simulink model "Winda_2015b"  (R2015b)
settings: Solver=FixedStepDiscrete  StartTime=0.0  StopTime=100  FixedStep=0.05  MaxStep=0.1  MinStep=0.01  RelTol=1e-3
undefined symbols (not defined in the file): sigbuilder_block
libraries: simulink x12
settings Model: Creator=dmar  LastModifiedBy=lab
settings DataIOCC: SaveFormat=Array  SignalLoggingSaveFormat=ModelDataLogs
settings OptimizationCC: ExpressionDepthLimit=2147483647
settings DebuggingCC: UnderspecifiedInitializationDetection=Classic  MergeDetectMultiDrivingBlocksExec=none  SolverPrmCheckMsg=warning  ParameterPrecisionLossMsg=none  FcnCallInpInsideContextMsg=UseLocalSettings  StateNameClashWarn=warning
settings HardwareCC: ProdBitPerPointer=32  ProdLargestAtomicFloat=None  ProdIntDivRoundTo=Undefined  ProdEndianess=Unspecified  ProdWordSize=32  ProdHWDeviceType=32-bit Generic
settings SFSimCC: SimParseCustomCode=off
settings GRTTargetCC: GeneratePreprocessorConditionals=Disable all  CombineOutputUpdateFcns=off  GRTInterface=on
settings ConfigComp: CovModelRefEnable=Off

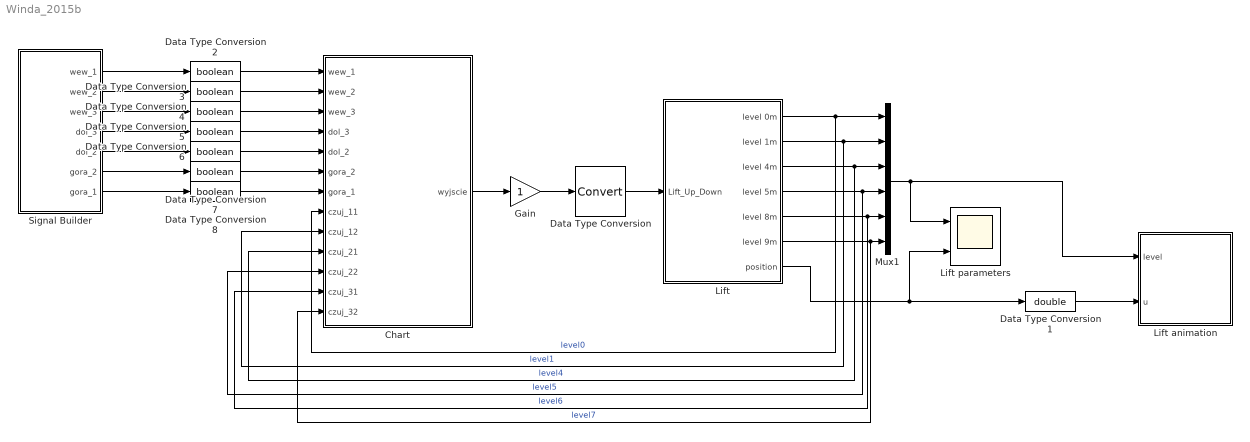
== system Winda_2015b ==
  Chart : Stateflow chart  TreatAsAtomicUnit=on
  Data Type Conversion : DataTypeConversion
  Data Type Conversion1 : DataTypeConversion  OutDataTypeStr=double
  Data Type Conversion{2..8} (7 alike) : DataTypeConversion  OutDataTypeStr=boolean
  Gain : Gain
  Lift : Subsystem
  Lift animation : MATLAB Function  TreatAsAtomicUnit=on  SystemSampleTime=0.05
  Lift parameters : Scope  NumInputPorts=2
  Mux1 : Mux  Inputs=6
  Signal Builder : Subsystem  Tag=STV Subsys  LoadFcn=sigbuilder_block('load',[81 111.75 550.5 630.75 ]);  StartFcn=sigbuilder_block('start');  StopFcn=sigbuilder_block('stop');  ClipboardFcn=sigbuilder_block('clipboard');  mask(Sigbuilder block){}
      mask help: Simulink:masks:SigbuilderBlock_MD
      mask init:
      | if ~strcmp(get_param(bdroot(gcbh),'SimulationStatus'),'stopped') tuvar = sigbuilder_block('maskInit'); end
      settings: CopyFcn=sigbuilder_block('copy');  DeleteFcn=sigbuilder_block('delete');  ModelCloseFcn=sigbuilder_block('modelClose');  PreSaveFcn=sigbuilder_block('preSave');  PauseFcn=sigbuilder_block('pause');  ContinueFcn=sigbuilder_block('continue');  NameChangeFcn=sigbuilder_block('namechange');  OpenFcn=sigbuilder_block('open',[81 111.75 550.5 630.75 ]);  CloseFcn=sigbuilder_block('close');
      mask Display: plot(0, 0, 100, 100,[2, 2, 32, 32, 2], [68, 8, 8, 68, 68],[32, 2], [38, 38], [32, 19, 2],[53, 60, 44], [32, 17, 17, 2],[16, 16, 31, 31]);txt = getActiveGroup(gcbh);text(2, 100, txt,'verticalAlignment', 'top');
  wires:
  Lift/7(position) -> Lift parameters/2, Data Type Conversion1/1
  Gain/1 -> Data Type Conversion/1
  Mux1/1 -> Lift parameters/1, Lift animation/1(level)
  Lift/1(level 0m) -> Chart/8(czuj_11), Mux1/1  "level0"
  Lift/2(level 1m) -> Chart/9(czuj_12), Mux1/2  "level1"
  Lift/3(level 4m) -> Chart/10(czuj_21), Mux1/3  "level4"
  Lift/4(level 5m) -> Chart/11(czuj_22), Mux1/4  "level5"
  Lift/5(level 8m) -> Mux1/5, Chart/12(czuj_31)  "level6"
  Lift/6(level 9m) -> Mux1/6, Chart/13(czuj_32)  "level7"
  Data Type Conversion/1 -> Lift/1(Lift_Up_Down)
  Data Type Conversion1/1 -> Lift animation/2(u)
  Chart/1(wyjscie) -> Gain/1
  Signal Builder/2(wew_2) -> Data Type Conversion3/1
  Signal Builder/3(wew_3) -> Data Type Conversion4/1
  Signal Builder/4(dol_3) -> Data Type Conversion5/1
  Signal Builder/5(dol_2) -> Data Type Conversion6/1
  Signal Builder/6(gora_2) -> Data Type Conversion7/1
  Signal Builder/7(gora_1) -> Data Type Conversion8/1
  Signal Builder/1(wew_1) -> Data Type Conversion2/1
  Data Type Conversion2/1 -> Chart/1(wew_1)
  Data Type Conversion3/1 -> Chart/2(wew_2)
  Data Type Conversion4/1 -> Chart/3(wew_3)
  Data Type Conversion5/1 -> Chart/4(dol_3)
  Data Type Conversion6/1 -> Chart/5(dol_2)
  Data Type Conversion7/1 -> Chart/6(gora_2)
  Data Type Conversion8/1 -> Chart/7(gora_1)

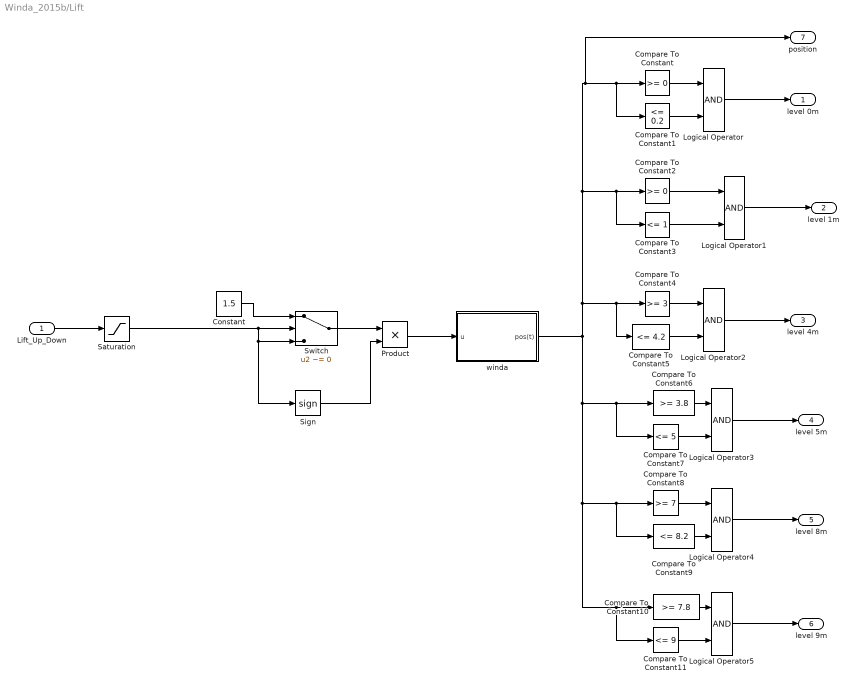
== system Winda_2015b/Lift ==
  Lift_Up_Down : Inport
  Compare To Constant : simulink/Logic and Bit Operations/Compare To Constant  relop=>=  const=0  OutDataTypeStr=boolean
  Compare To Constant1 : simulink/Logic and Bit Operations/Compare To Constant  relop=<=  const=0.2  OutDataTypeStr=boolean
  Compare To Constant10 : simulink/Logic and Bit Operations/Compare To Constant  relop=>=  const=7.8  OutDataTypeStr=boolean
  Compare To Constant11 : simulink/Logic and Bit Operations/Compare To Constant  relop=<=  const=9  OutDataTypeStr=boolean
  Compare To Constant2 : simulink/Logic and Bit Operations/Compare To Constant  relop=>=  const=0  OutDataTypeStr=boolean
  Compare To Constant3 : simulink/Logic and Bit Operations/Compare To Constant  relop=<=  const=1  OutDataTypeStr=boolean
  Compare To Constant4 : simulink/Logic and Bit Operations/Compare To Constant  relop=>=  const=3  OutDataTypeStr=boolean
  Compare To Constant5 : simulink/Logic and Bit Operations/Compare To Constant  relop=<=  const=4.2  OutDataTypeStr=boolean
  Compare To Constant6 : simulink/Logic and Bit Operations/Compare To Constant  relop=>=  const=3.8  OutDataTypeStr=boolean
  Compare To Constant7 : simulink/Logic and Bit Operations/Compare To Constant  relop=<=  const=5  OutDataTypeStr=boolean
  Compare To Constant8 : simulink/Logic and Bit Operations/Compare To Constant  relop=>=  const=7  OutDataTypeStr=boolean
  Compare To Constant9 : simulink/Logic and Bit Operations/Compare To Constant  relop=<=  const=8.2  OutDataTypeStr=boolean
  Constant : Constant  Value=1.5
  Logical Operator{,1..5} (6 alike) : Logic  AllPortsSameDT=off  OutDataTypeStr=boolean
  Product : Product  OutDataTypeStr=Inherit: Inherit via back propagation  RndMeth=Zero
  Saturation : Saturate  UpperLimit=1  LowerLimit=-1
  Sign : Signum
  Switch : Switch  Criteria=u2 ~= 0  OutDataTypeStr=Inherit: Inherit via back propagation
  winda : Subsystem
  level 0m : Outport
  level 1m : Outport  Port=2
  level 4m : Outport  Port=3
  level 5m : Outport  Port=4
  level 8m : Outport  Port=5
  level 9m : Outport  Port=6
  position : Outport  Port=7
  wires:
  Constant/1 -> Switch/1
  Lift_Up_Down/1 -> Saturation/1
  Switch/1 -> Product/1
  Product/1 -> winda/1(u)
  Sign/1 -> Product/2
  Logical Operator/1 -> level 0m/1
  Compare To Constant/1 -> Logical Operator/1
  Compare To Constant1/1 -> Logical Operator/2
  Logical Operator1/1 -> level 1m/1
  Compare To Constant2/1 -> Logical Operator1/1
  Compare To Constant3/1 -> Logical Operator1/2
  Logical Operator2/1 -> level 4m/1
  Compare To Constant4/1 -> Logical Operator2/1
  Compare To Constant5/1 -> Logical Operator2/2
  Logical Operator3/1 -> level 5m/1
  Compare To Constant6/1 -> Logical Operator3/1
  Compare To Constant7/1 -> Logical Operator3/2
  Logical Operator4/1 -> level 8m/1
  Compare To Constant8/1 -> Logical Operator4/1
  Compare To Constant9/1 -> Logical Operator4/2
  Logical Operator5/1 -> level 9m/1
  winda/1(pos(t)) -> position/1, Compare To Constant1/1, Compare To Constant/1, Compare To Constant2/1, Compare To Constant3/1, Compare To Constant5/1, Compare To Constant4/1, Compare To Constant10/1, Compare To Constant11/1, Compare To Constant9/1, Compare To Constant8/1, Compare To Constant6/1, Compare To Constant7/1
  Compare To Constant10/1 -> Logical Operator5/1
  Compare To Constant11/1 -> Logical Operator5/2
  Saturation/1 -> Sign/1, Switch/3, Switch/2

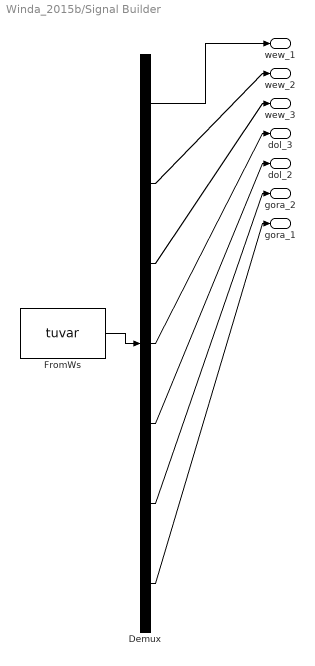
== system Winda_2015b/Signal Builder ==
  Demux : Demux  Tag=STV Demux  Outputs=7
  FromWs : FromWorkspace  Tag=STV FromWs  VariableName=tuvar  SampleTime=0
      SigBuilderData=|
      | common.afterFinalStr = 'Extrapolate'
      | common.sampleTime = 0
      | dataSet(1).timeRange = [0 100]
      | dataSet(1).name = 'Bazowanie'
      | dataSet(2).timeRange = [0 100]
      | dataSet(2).name = 'Test1'
      | dataSet(3).timeRange = [0 100]
      | dataSet(3).name = 'Test2'
      | dataSet(4).timeRange = [0 100]
      | dataSet(4).name = 'Test3'
      | dataSet(5).timeRange = [0 100]
      | dataSet(5).name = 'patologia'
      | sbobj.Groups(1).Name = 'Bazowanie'
      | sbobj.Groups(1).Signals(1).Name = 'wew_1'
      | sbobj.Groups(1).Signals(1).XData = [0 15.3 19.1 26.7 100]
      | sbobj.Groups(1).Signals(1).YData = [0 0 0 0 0]
      | sbobj.Groups(1).Signals(2).Name = 'wew_2'
      | sbobj.Groups(1).Signals(2).XData = [0 4.9 4.9 9.9 9.9 100]
      | sbobj.Groups(1).Signals(2).YData = [0 0 1 1 0 0]
      | sbobj.Groups(1).Signals(3).Name = 'wew_3'
      | sbobj.Groups(1).Signals(3).XData = [0 16 24 100]
      | sbobj.Groups(1).Signals(3).YData = [0 0 0 0]
      | sbobj.Groups(1).Signals(4).Name = 'dol_3'
      | sbobj.Groups(1).Signals(4).XData = [0 20 20 25 25 100]
      | sbobj.Groups(1).Signals(4).YData = [0 0 1 1 0 0]
      | sbobj.Groups(1).Signals(5).Name = 'dol_2'
      | sbobj.Groups(1).Signals(5).XData = [0 40.8 40.8 45.8 45.8 100]
      | sbobj.Groups(1).Signals(5).YData = [0 0 1 1 0 0]
      | sbobj.Groups(1).Signals(6).Name = 'gora_2'
      | sbobj.Groups(1).Signals(6).XData = [0 5.01 9 100]
      | sbobj.Groups(1).Signals(6).YData = [0 0 0 0]
      | sbobj.Groups(1).Signals(7).Name = 'gora_1'
      | sbobj.Groups(1).Signals(7).XData = [0 16 24 100]
      | sbobj.Groups(1).Signals(7).YData = [0 0 0 0]
      | sbobj.Groups(1).TimeRange = [0 100]
      | sbobj.Groups(2).Name = 'Test1'
      | sbobj.Groups(2).Signals(1).Name = 'wew_1'
      | sbobj.Groups(2).Signals(1).XData = [0 22.6 22.6 26.7 26.7 100]
      | sbobj.Groups(2).Signals(1).YData = [0 0 1 1 0 0]
      | sbobj.Groups(2).Signals(2).Name = 'wew_2'
      | sbobj.Groups(2).Signals(2).XData = [0 4.9 4.9 7.6 7.6 100]
      | sbobj.Groups(2).Signals(2).YData = [0 0 1 1 0 0]
      | sbobj.Groups(2).Signals(3).Name = 'wew_3'
      | sbobj.Groups(2).Signals(3).XData = [0 45.4 51 100]
      | sbobj.Groups(2).Signals(3).YData = [0 0 0 0]
      | sbobj.Groups(2).Signals(4).Name = 'dol_3'
      | sbobj.Groups(2).Signals(4).XData = [0 17.4 17.4 20 20 100]
      | sbobj.Groups(2).Signals(4).YData = [0 0 1 1 0 0]
      | sbobj.Groups(2).Signals(5).Name = 'dol_2'
      | sbobj.Groups(2).Signals(5).XData = [0 26 28.3 100]
      | sbobj.Groups(2).Signals(5).YData = [0 0 0 0]
      | sbobj.Groups(2).Signals(6).Name = 'gora_2'
      | sbobj.Groups(2).Signals(6).XData = [0 50 50 59 59 100]
      | sbobj.Groups(2).Signals(6).YData = [0 0 1 1 0 0]
      | sbobj.Groups(2).Signals(7).Name = 'gora_1'
      | sbobj.Groups(2).Signals(7).XData = [0 16 24 100]
      | sbobj.Groups(2).Signals(7).YData = [0 0 0 0]
      | sbobj.Groups(2).TimeRange = [0 100]
      | sbobj.Groups(3).Name = 'Test2'
      | sbobj.Groups(3).Signals(1).Name = 'wew_1'
      | sbobj.Groups(3).Signals(1).XData = [0 22.6 26.7 100]
      | sbobj.Groups(3).Signals(1).YData = [0 0 0 0]
      | sbobj.Groups(3).Signals(2).Name = 'wew_2'
      | sbobj.Groups(3).Signals(2).XData = [0 4.9 4.9 7.6 7.6 100]
      | sbobj.Groups(3).Signals(2).YData = [0 0 1 1 0 0]
      | sbobj.Groups(3).Signals(3).Name = 'wew_3'
      | sbobj.Groups(3).Signals(3).XData = [0 30.4 30.4 40 40 100]
      | sbobj.Groups(3).Signals(3).YData = [0 0 1 1 0 0]
      | sbobj.Groups(3).Signals(4).Name = 'dol_3'
      | sbobj.Groups(3).Signals(4).XData = [0 17.4 20 100]
      | sbobj.Groups(3).Signals(4).YData = [0 0 0 0]
      | sbobj.Groups(3).Signals(5).Name = 'dol_2'
      | sbobj.Groups(3).Signals(5).XData = [0 45.8 45.8 49.6 49.6 100]
      | sbobj.Groups(3).Signals(5).YData = [0 0 1 1 0 0]
      | sbobj.Groups(3).Signals(6).Name = 'gora_2'
      | sbobj.Groups(3).Signals(6).XData = [0 50 59 100]
      | sbobj.Groups(3).Signals(6).YData = [0 0 0 0]
      | sbobj.Groups(3).Signals(7).Name = 'gora_1'
      | sbobj.Groups(3).Signals(7).XData = [0 16.4 16.4 20.8 20.8 100]
      | sbobj.Groups(3).Signals(7).YData = [0 0 1 1 0 0]
      | sbobj.Groups(3).TimeRange = [0 100]
      | sbobj.Groups(4).Name = 'Test3'
      | sbobj.Groups(4).Signals(1).Name = 'wew_1'
      | sbobj.Groups(4).Signals(1).XData = [0 22.6 26.7 100]
      | sbobj.Groups(4).Signals(1).YData = [0 0 0 0]
      | sbobj.Groups(4).Signals(2).Name = 'wew_2'
      | sbobj.Groups(4).Signals(2).XData = [0 76.8 76.8 86.2 86.2 100]
      | sbobj.Groups(4).Signals(2).YData = [0 0 1 1 0 0]
      | sbobj.Groups(4).Signals(3).Name = 'wew_3'
      | sbobj.Groups(4).Signals(3).XData = [0 9.4 9.4 15.4 15.4 100]
      | sbobj.Groups(4).Signals(3).YData = [0 0 1 1 0 0]
      | sbobj.Groups(4).Signals(4).Name = 'dol_3'
      | sbobj.Groups(4).Signals(4).XData = [0 17.4 20 100]
      | sbobj.Groups(4).Signals(4).YData = [0 0 0 0]
      | sbobj.Groups(4).Signals(5).Name = 'dol_2'
      | sbobj.Groups(4).Signals(5).XData = [0 10.4 10.4 24.4 24.4 100]
      | sbobj.Groups(4).Signals(5).YData = [0 0 1 1 0 0]
      | sbobj.Groups(4).Signals(6).Name = 'gora_2'
      | sbobj.Groups(4).Signals(6).XData = [0 50 59 100]
      | sbobj.Groups(4).Signals(6).YData = [0 0 0 0]
      | sbobj.Groups(4).Signals(7).Name = 'gora_1'
      | sbobj.Groups(4).Signals(7).XData = [0 77 77 83.6 83.6 100]
      | sbobj.Groups(4).Signals(7).YData = [0 0 1 1 0 0]
      | sbobj.Groups(4).TimeRange = [0 100]
      | sbobj.Groups(5).Name = 'patologia'
      | sbobj.Groups(5).Signals(1).Name = 'wew_1'
      | sbobj.Groups(5).Signals(1).XData = [0 40.6 40.6 51.8 51.8 100]
      | sbobj.Groups(5).Signals(1).YData = [0 0 1 1 0 0]
      | sbobj.Groups(5).Signals(2).Name = 'wew_2'
      | sbobj.Groups(5).Signals(2).XData = [0 80 80 85.4 85.4 100]
      | sbobj.Groups(5).Signals(2).YData = [0 0 1 1 0 0]
      | sbobj.Groups(5).Signals(3).Name = 'wew_3'
      | sbobj.Groups(5).Signals(3).XData = [0 10 10 15.4 15.4 100]
      | sbobj.Groups(5).Signals(3).YData = [0 0 1 1 0 0]
      | sbobj.Groups(5).Signals(4).Name = 'dol_3'
      | sbobj.Groups(5).Signals(4).XData = [0 19.4 19.4 41.4 41.4 100]
      | sbobj.Groups(5).Signals(4).YData = [0 0 1 1 0 0]
      | sbobj.Groups(5).Signals(5).Name = 'dol_2'
      | sbobj.Groups(5).Signals(5).XData = [0 20.8 20.8 24.6 24.6 100]
      | sbobj.Groups(5).Signals(5).YData = [0 0 1 1 0 0]
      | sbobj.Groups(5).Signals(6).Name = 'gora_2'
      | sbobj.Groups(5).Signals(6).XData = [0 47.2 59 100]
      | sbobj.Groups(5).Signals(6).YData = [0 0 0 0]
      | sbobj.Groups(5).Signals(7).Name = 'gora_1'
      | sbobj.Groups(5).Signals(7).XData = [0 18.4 18.4 32.2 32.2 100]
      | sbobj.Groups(5).Signals(7).YData = [0 0 1 1 0 0]
      | sbobj.Groups(5).TimeRange = [0 100]
  wew_1 : Outport  Tag=STV Outport
  wew_2 : Outport  Tag=STV Outport  Port=2
  wew_3 : Outport  Tag=STV Outport  Port=3
  dol_3 : Outport  Tag=STV Outport  Port=4
  dol_2 : Outport  Tag=STV Outport  Port=5
  gora_2 : Outport  Tag=STV Outport  Port=6
  gora_1 : Outport  Tag=STV Outport  Port=7
  wires:
  Demux/1 -> wew_1/1
  FromWs/1 -> Demux/1
  Demux/2 -> wew_2/1
  Demux/3 -> wew_3/1
  Demux/4 -> dol_3/1
  Demux/5 -> dol_2/1
  Demux/6 -> gora_2/1
  Demux/7 -> gora_1/1

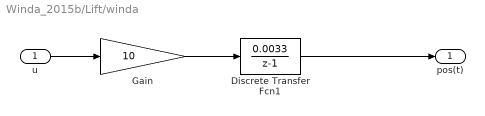
== system Winda_2015b/Lift/winda ==
  u : Inport
  Discrete Transfer Fcn1 : DiscreteTransferFcn  Numerator=[0.0033]  Denominator=[1 -1]  SampleTime=0.05  StateDataTypeStr=fixdt(1,26,12)  NumCoefDataTypeStr=fixdt(1,26,12)  DenCoefDataTypeStr=fixdt(1,26,12)  NumProductDataTypeStr=fixdt(1,26,12)  DenProductDataTypeStr=fixdt(1,26,12)  NumAccumDataTypeStr=fixdt(1,26,12)  DenAccumDataTypeStr=fixdt(1,26,12)  OutDataTypeStr=fixdt(1,26,12)
  Gain : Gain  Gain=10  ParamDataTypeStr=fixdt(1,15,2)  OutDataTypeStr=Inherit: Same as input
  pos(t) : Outport
  wires:
  u/1 -> Gain/1
  Gain/1 -> Discrete Transfer Fcn1/1
  Discrete Transfer Fcn1/1 -> pos(t)/1

== matlab function Winda_2015b/Lift animation ==
  data: level input; u input
function plot_Lift3( level,u)
%#codegen




persistent fig3;
persistent NOWE1;
persistent L_pos;


if isempty(L_pos),

    if isempty(fig3), 
    fig3 = figure(3);
    else
    close(fig3);
    fig3 = figure(3);
    end
     %NOWE1 = [0 0.1 0.1 0 0; 0.25 .25 0 0 .25]*10;
    NOWE1 = [.1 0 0 .1 .1 .09 .09 .1; 0 0 0.25 0.25 0 0 0.12 .12]*10;
    
    axis([-4 4 -1 15]);
    grid('off');
    %xlabel('X position [m]');
    ylabel('Lift position [m]');
    hold('on');
    line([-0.05 -0.05],[0 12],'LineWidth',2,'Color','k')
    line([1.05 1.05],[0 12],'LineWidth',2,'Color','k')
    line([-4 4],[-0.05 -0.05],'LineWidth',2,'Color','k')
    
    line([-1 -0.05],[4 4],'LineWidth',2,'Color','k')
    line([1.05 2],[4 4],'LineWidth',2,'Color','k')
    
    line([-1 -0.05],[8 8],'LineWidth',2,'Color','k')
    line([1.05 2],[8 8],'LineWidth',2,'Color','k')
    
    line([-1 -0.05],[12 12],'LineWidth',2,'Color','k')
    line([1.05 2],[12 12],'LineWidth',2,'Color','k')
    
 % czarna lampka na wysokosci 0
 line([1.05 1.2],[0.2 0.2],'LineWidth',4,'Color','k')

 % czarna lampka na wysokosci 1
 line([1.05 1.2],[1 1],'LineWidth',4,'Color','k')
    
 % czarna lampka na wysokosci 4
 line([1.05 1.2],[4 4],'LineWidth',4,'Color','k')

 % czarna lampka na wysokosci 5
 line([1.05 1.2],[5 5],'LineWidth',4,'Color','k')
    
  % czarna lampka na wysokosci 8
 line([1.05 1.2],[8 8],'LineWidth',4,'Color','k')
 % czarna lampka na wysokosci 9
 line([1.05 1.2],[9 9],'LineWidth',4,'Color','k')
   
%plot(NOWE1(1,:),NOWE1(2,:)+prev1,'w');
L_pos=plot(NOWE1(1,:),NOWE1(2,:)+u,'b');
    
    
    
else
    if(ishghandle(L_pos)),
       
        set(L_pos,'yData',NOWE1(2,:)+u);


if level(1)==1    
 % czarna lampka na wysokosci 0
 line([1.05 1.2],[0.2 0.2],'LineWidth',4,'Color','r');
else
 line([1.05 1.2],[0.2 0.2],'LineWidth',4,'Color','k');
end

if level(2)==1    
 % czarna lampka na wysokosci 1
 line([1.05 1.2],[1 1],'LineWidth',4,'Color','r');
else
 line([1.05 1.2],[1 1],'LineWidth',4,'Color','k');
end

if level(3)==1    
 % czarna lampka na wysokosci 4
 line([1.05 1.2],[4 4],'LineWidth',4,'Color','r');
else
 line([1.05 1.2],[4 4],'LineWidth',4,'Color','k');
end

if level(4)==1    
 % czarna lampka na wysokosci 5
 line([1.05 1.2],[5 5],'LineWidth',4,'Color','r');
else
 line([1.05 1.2],[5 5],'LineWidth',4,'Color','k');
end

if level(5)==1    
 % czarna lampka na wysokosci 8
 line([1.05 1.2],[8 8],'LineWidth',4,'Color','r');
else
 line([1.05 1.2],[8 8],'LineWidth',4,'Color','k');
end

if level(6)==1    
 % czarna lampka na wysokosci 9
 line([1.05 1.2],[9 9],'LineWidth',4,'Color','r');
else
 line([1.05 1.2],[9 9],'LineWidth',4,'Color','k');
end



     
        
        
        
    end,
end

== stateflow chart Winda_2015b/Chart ==
  state poziom_1
    en: wyjscie=0;
  state w_gore_13
    en: wyjscie=1;
  state w_dol_21
    en: wyjscie=-1;
  state w_gore_12
    en: wyjscie=1;
  state poziom_2
    en: wyjscie=0;
  state zatrzymanie_2_gora
    en: wyjscie=0;
  state zatrzymanie_2_dol1
    en: wyjscie=0;
  state w_dol_32
    en: wyjscie=-1;
  state w_gore_23
    en: wyjscie=1;
  state poziom_3
    en: wyjscie=0;
  state w_dol_31
    en: wyjscie=-1;
  (default) -> poziom_1
  w_dol_31 -> poziom_1 [order 2] : [czuj_11==1 && czuj_12==1]
  poziom_1 -> w_gore_13 [order 2] : [wew_3==1 || dol_3==1]
  w_gore_13 -> poziom_3 [order 2] : [czuj_31==1 && czuj_32==1]
  w_dol_21 -> poziom_1 : [czuj_11==1 && czuj_12==1]
  poziom_1 -> w_gore_12 [order 1] : [wew_2==1 || gora_2==1 || dol_2==1]
  w_gore_13 -> zatrzymanie_2_gora [order 1] : [czuj_21==1 && czuj_22==1 && gora_2==1]
  zatrzymanie_2_dol1 -> w_dol_21 : [czuj_21==1 && czuj_22==1]
  poziom_2 -> w_dol_21 [order 3] : after(10,sec)
  w_gore_12 -> poziom_2 : [czuj_21==1 && czuj_22==1]
  poziom_2 -> w_dol_21 [order 1] : [wew_1==1 || gora_1==1 ]
  w_dol_32 -> poziom_2 : [czuj_21==1 && czuj_22==1]
  poziom_2 -> w_gore_23 [order 2] : [wew_3==1 || dol_3==1]
  w_dol_31 -> zatrzymanie_2_dol1 [order 1] : [czuj_21==1 && czuj_22==1 && dol_2==1]
  zatrzymanie_2_gora -> w_gore_23 : [czuj_21==1 && czuj_22==1]
  w_gore_23 -> poziom_3 : [czuj_31==1 && czuj_32==1]
  poziom_3 -> w_dol_32 [order 1] : [wew_2==1 || gora_2==1 || dol_2==1]
  poziom_3 -> w_dol_31 [order 2] : [wew_1==1 || gora_1==1]
  poziom_3 -> w_dol_31 [order 3] : after(10,sec)
  data: wew_1 input boolean; wew_2 input boolean; wew_3 input boolean; dol_3 input boolean; dol_2 input boolean; gora_2 input boolean; gora_1 input boolean; wyjscie output double; czuj_11 input boolean; czuj_12 input boolean; czuj_21 input boolean; czuj_22 input boolean; czuj_31 input boolean; czuj_32 input boolean
